simulink model "hardware"  (R2018a)
settings: Solver=VariableStepDiscrete  StartTime=0.0  StopTime=0.1  RelTol=1e-3
libraries: powerlib x17
settings Model: Creator=ekoma  LastModifiedBy=Onur

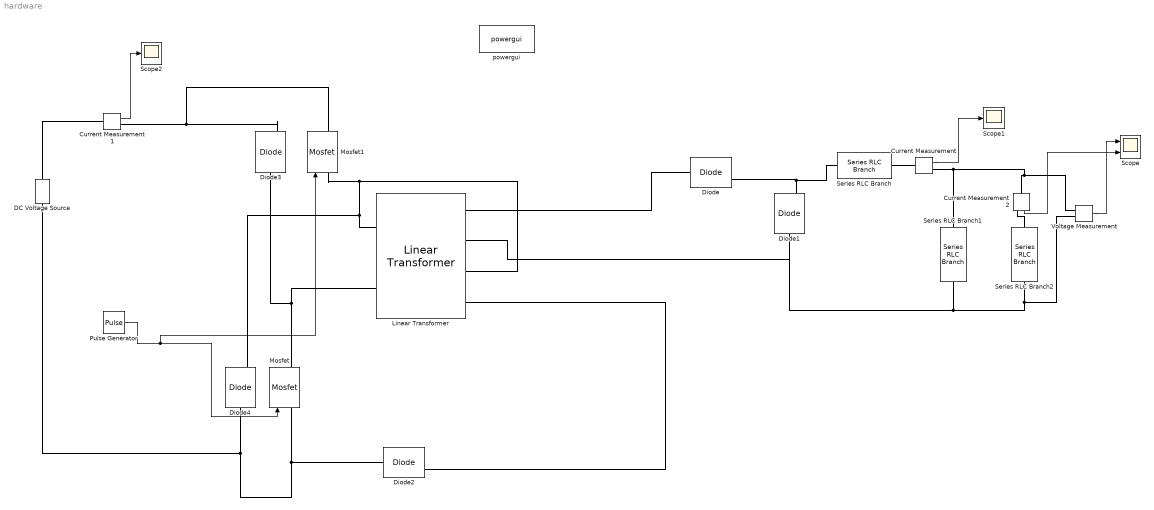
== system hardware ==
  Current Measurement : powerlib/Measurements/Current Measurement  PhasorSimulation=off  OutputType=Complex  PSBequivalent=0
  Current Measurement1 : powerlib/Measurements/Current Measurement  PhasorSimulation=off  OutputType=Complex  PSBequivalent=0
  Current Measurement2 : powerlib/Measurements/Current Measurement  PhasorSimulation=off  OutputType=Complex  PSBequivalent=0
  DC Voltage Source : powerlib/Electrical Sources/DC Voltage Source  Amplitude=48  Measurements=None
  Diode{,1,3..4} (4 alike) : powerlib/Power Electronics/Diode  Ron=0.001  Lon=0  Vf=0.7  IC=0  UseSnubber=0  Rs=500  Cs=250e-9  Measurements=on
  Diode2 : powerlib/Power Electronics/Diode  Ron=0.001  Lon=0  Vf=0.8  IC=0  UseSnubber=0  Rs=500  Cs=250e-9  Measurements=on
  Linear Transformer : powerlib/Elements/Linear Transformer  UNITS=SI  NominalPower=[ 40 32000 ]  winding1=[16 0.080 1.65e-6]  winding2=[20 0.080 1.65e-6]  ThreeWindings=on  winding3=[16 0.080 1.65e-6]  RmLm=[1.0805e+06 71.2e-6]  Measurements=All voltages and currents  DataType=on
  Mosfet : powerlib/Power Electronics/Mosfet  Ron=0.1  Lon=0  Rd=0.01  Vfd=10000  IC=0  Rs=1e5  Cs=inf  Measurements=on
  Mosfet1 : powerlib/Power Electronics/Mosfet  Ron=0.1  Lon=0  Rd=0.01  Vfd=10000  IC=0  Rs=1e5  Cs=inf  Measurements=on
  Pulse Generator : DiscretePulseGenerator  PulseType=Time based  Amplitude=5  Period=1/32000  PulseWidth=20
  Scope : Scope  NumInputPorts=2
  Scope1 : Scope
  Scope2 : Scope
  Series RLC Branch : powerlib/Elements/Series RLC Branch  LConnTagsString=__new0  RConnTagsString=__new0  BranchType=L  Resistance=1  Inductance=2.2e-3  SetiL0=off  InitialCurrent=0  Capacitance=1e-6  Setx0=off  InitialVoltage=0  Measurements=None
  Series RLC Branch1 : powerlib/Elements/Series RLC Branch  LConnTagsString=__new0  RConnTagsString=__new0  BranchType=C  Resistance=1  Inductance=1e-3  SetiL0=off  InitialCurrent=0  Capacitance=47e-6  Setx0=off  InitialVoltage=0  Measurements=None
  Series RLC Branch2 : powerlib/Elements/Series RLC Branch  LConnTagsString=__new0  RConnTagsString=__new0  BranchType=R  Resistance=2.5  Inductance=1e-3  SetiL0=off  InitialCurrent=0  Capacitance=1e-6  Setx0=off  InitialVoltage=0  Measurements=None
  Voltage Measurement : powerlib/Measurements/Voltage Measurement  PhasorSimulation=off  OutputType=Complex  PSBequivalent=0
  powergui : powerlib/powergui  Priority=1  SimulationMode=Discrete  SampleTime=2e-7  frequency=60  Iterations=50  frequencyindice=0  Pbase=100e6  ErrMax=1e-4  UnitsV=kV  UnitsW=MW  buscounter=0  FunctionMessages=off  echomessages=off  EnableUseOfTLC=off  CurrentSourceSwitches=off  DisableSnubberDevices=off  DisableRonSwitches=off  DisableVfSwitches=off  DisplayEquations=off  SolverType=Tustin/Backward Euler (TBE)  Interpol=off  ExternalGateDelay=off  methode=off  Ts=100  x0status=blocks  SPID=on  SwTol=0  HookPort=off  RestoreLinks=warning  ResistiveCurrentMeasurement=off  Frange=[0:2:500]  Ylog=off  Xlog=on  ShowGrid=off  save=off  variable=ZData  structure=0  ZoomFFT=off  StartTime=0.0  cycles=1  DisplayStyle=1  fundamental=60  FreqAxis=off  MaxFrequency=1000  frequencyindicesteady=1  RmsSteady=1  display=off
  wires:
  Pulse Generator/1 -> Mosfet1/1, Mosfet/1
  Voltage Measurement/1 -> Scope/1
  Current Measurement/1 -> Scope1/1
  Current Measurement1/1 -> Scope2/1
  Current Measurement2/1 -> Scope/2
  connections:
  Diode/LConn1 -- Linear Transformer/RConn1
  Diode/RConn1 -- Series RLC Branch/LConn1 -- Diode1/RConn1
  Current Measurement/LConn1 -- Series RLC Branch/RConn1
  Voltage Measurement/LConn1 -- Current Measurement2/LConn1 -- Series RLC Branch1/LConn1 -- Current Measurement/RConn1
  Linear Transformer/LConn1 -- Diode4/RConn1 -- Linear Transformer/RConn3 -- Mosfet1/LConn1
  Series RLC Branch2/RConn1 -- Voltage Measurement/LConn2 -- Series RLC Branch1/RConn1 -- Linear Transformer/RConn2 -- Diode1/LConn1
  Diode2/RConn1 -- Linear Transformer/RConn4
  Mosfet/RConn1 -- Diode3/LConn1 -- Linear Transformer/LConn2
  DC Voltage Source/LConn1 -- Mosfet/LConn1 -- Diode2/LConn1 -- Diode4/LConn1
  Current Measurement1/LConn1 -- DC Voltage Source/RConn1
  Mosfet1/RConn1 -- Current Measurement1/RConn1 -- Diode3/RConn1
  Series RLC Branch2/LConn1 -- Current Measurement2/RConn1
